simulink model "stateFlowFunctions"  (R2024a)
settings: Solver=FixedStepDiscrete  StartTime=0.0  StopTime=10.0  FixedStep=.1  RelTol=1e-3
settings Model: Creator=User  LastModifiedBy=User

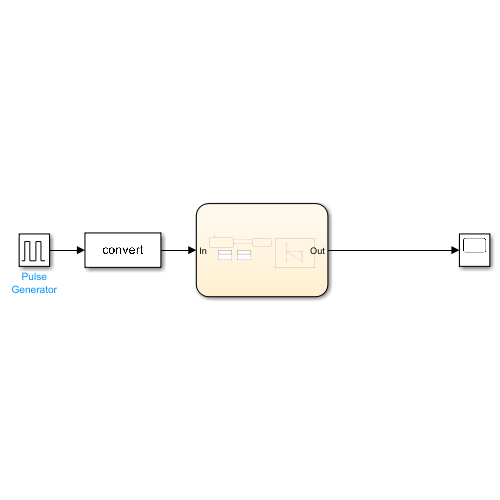
[thumbnail: Simulink's stored preview of the top-level diagram]
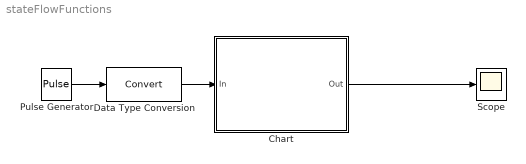
== system stateFlowFunctions ==
  Chart : Stateflow chart  TreatAsAtomicUnit=on
  Data Type Conversion : DataTypeConversion  SaturateOnIntegerOverflow=off  RndMeth=Floor
  Pulse Generator : DiscretePulseGenerator  PulseType=Time based  Period=10  PulseWidth=5
  Scope : Scope
  wires:
  Data Type Conversion/1 -> Chart/1(In)
  Pulse Generator/1 -> Data Type Conversion/1
  Chart/1(Out) -> Scope/1

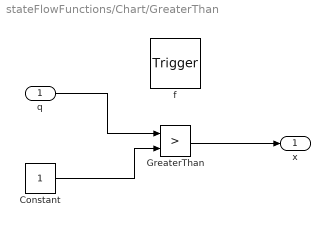
== system stateFlowFunctions/Chart/GreaterThan ==
  q : Inport  OutDataTypeStr=double  PortDimensions=1
  f : TriggerPort  TriggerType=function-call  VariantControl=(inherit)
      settings: CopyFcn=Stateflow.SLINSF.SimulinkMan.removeBlockPreDeleteFcn  PreDeleteFcn=Stateflow.SLINSF.SimulinkMan.unsafePredeleteFcn
  Constant : Constant
  GreaterThan : RelationalOperator  Operator=>  OutDataTypeStr=boolean  RndMeth=Simplest  InputSameDT=off
  x : Outport  OutDataTypeStr=boolean
  wires:
  q/1 -> GreaterThan/1
  Constant/1 -> GreaterThan/2
  GreaterThan/1 -> x/1

== stateflow chart stateFlowFunctions/Chart ==
  state ON_State
    Local_var=GreaterThan(In);
    Local_var2=calcFact(5);
  state OFF_State
    local_SQRT=theSqrt(In);
  state x=calcFact(q) [function]
    (default) -> (junction 28) : /* calculation of Factorial */
    (junction 28) -> (junction 30) : {index=q;x=1;}
    (junction 30) -> (junction 29) [order 1] : [index > 0]
    (junction 32) -> (junction 30)
    (junction 30) -> (junction 33) [order 2]
    (junction 29) -> (junction 31)
    (junction 31) -> (junction 32) : {
        | x=x*index;
        | index--;
        | }
  state x=GreaterThan(q) [function]
  (default) -> ON_State
  ON_State -> OFF_State : [Local_var]
  OFF_State -> ON_State
  data: q function_input double; x function_output double; q function_input double size=1; x function_output boolean; q function_input double; x function_output double; In input boolean; Out output uint8; Local_var local boolean =0; local_SQRT local double =0; index local double =0; Local_var2 local double =0
  function x=theSqrt(q):
    | function x=theSqrt(q)
    | x=sqrt(q);
    | end
